simulink model "simulation_avion_complet_naturel"  (R2019b)
settings: Solver=VariableStepAuto  StartTime=0.0  StopTime=tsim  RelTol=1e-3
undefined symbols (not defined in the file): A_simp, B_simp, C_simp, D_simp
settings Model: Creator=natha  LastModifiedBy=natha

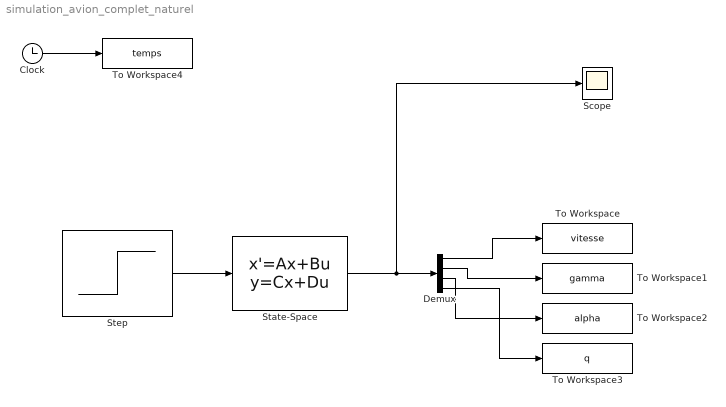
== system simulation_avion_complet_naturel ==
  Clock : Clock
  Demux : Demux
  Scope : Scope
  State-Space : StateSpace  A=A_simp  B=B_simp  C=C_simp  D=D_simp  InitialCondition=0
  Step : Step  Before=1  SampleTime=0
  To Workspace : ToWorkspace  VariableName=vitesse  SampleTime=-1
  To Workspace1 : ToWorkspace  VariableName=gamma  SampleTime=-1
  To Workspace2 : ToWorkspace  VariableName=alpha  SampleTime=-1
  To Workspace3 : ToWorkspace  VariableName=q  SampleTime=-1
  To Workspace4 : ToWorkspace  VariableName=temps  SampleTime=-1
  wires:
  Step/1 -> State-Space/1
  State-Space/1 -> Scope/1, Demux/1
  Demux/1 -> To Workspace/1
  Demux/2 -> To Workspace1/1
  Demux/3 -> To Workspace2/1
  Demux/4 -> To Workspace3/1
  Clock/1 -> To Workspace4/1
